simulink model "roll_loop"  (R2019a)
settings: Solver=VariableStepAuto  StartTime=0.0  StopTime=1000  RelTol=1e-3
undefined symbols (not defined in the file): AP, trans_func
settings Model: Creator=nikhil  LastModifiedBy=VTOL_HYD

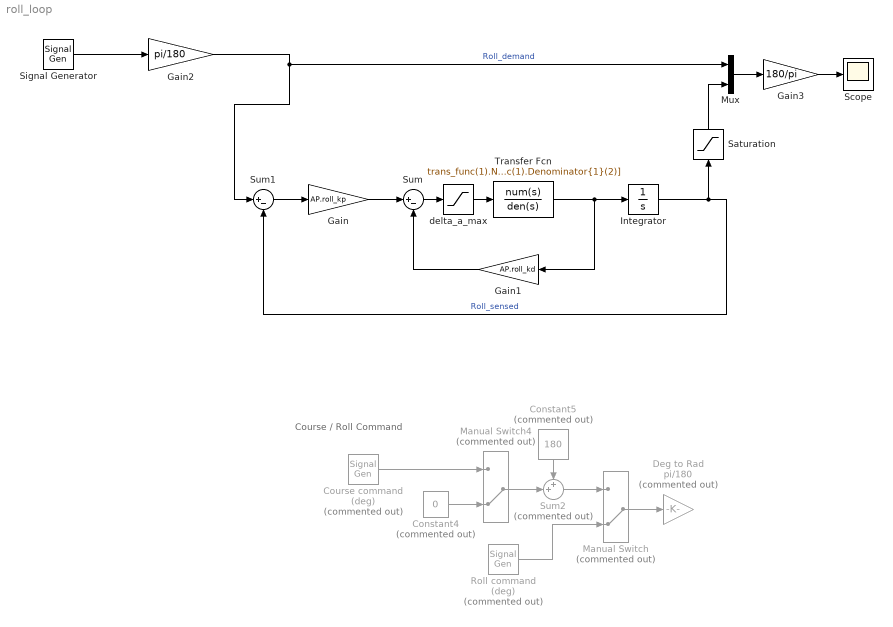
== system roll_loop ==
  note: Course / Roll Command
  Constant4 : Constant  Commented=on  Value=0
  Constant5 : Constant  Commented=on  Value=180
  Course command (deg) : SignalGenerator  Commented=on  WaveForm=square  Amplitude=45  Frequency=.02
  Deg to Rad : Gain  Commented=on  Gain=pi/180
  Gain : Gain  Gain=AP.roll_kp
  Gain1 : Gain  Gain=AP.roll_kd
  Gain2 : Gain  Gain=pi/180
  Gain3 : Gain  Gain=180/pi
  Integrator : Integrator
  Manual Switch : ManualSwitch  Commented=on  CurrentSetting=0
  Manual Switch4 : ManualSwitch  Commented=on  CurrentSetting=0
  Mux : Mux  Inputs=2
  Roll command (deg) : SignalGenerator  Commented=on  Amplitude=180  Frequency=0.1
  Saturation : Saturate  UpperLimit=7  LowerLimit=-7
  Scope : Scope
  Signal Generator : SignalGenerator  Amplitude=45  Frequency=.1  Units=rad/sec
  Sum : Sum  Inputs=|+-
  Sum1 : Sum  Inputs=|+-
  Sum2 : Sum  Commented=on  Inputs=++|
  Transfer Fcn : TransferFcn  Numerator=trans_func(1).Numerator{1}  Denominator=[trans_func(1).Denominator{1}(1), trans_func(1).Denominator{1}(2)]
  delta_a_max : Saturate  UpperLimit=0.785  LowerLimit=-.785
  wires:
  Transfer Fcn/1 -> Gain1/1, Integrator/1
  Integrator/1 -> Sum1/2, Saturation/1  "Roll_sensed"
  Gain1/1 -> Sum/2
  Gain2/1 -> Sum1/1, Mux/1  "Roll_demand"
  Sum1/1 -> Gain/1
  Gain/1 -> Sum/1
  Saturation/1 -> Mux/2
  Signal Generator/1 -> Gain2/1
  Mux/1 -> Gain3/1
  Gain3/1 -> Scope/1
  Sum/1 -> delta_a_max/1
  delta_a_max/1 -> Transfer Fcn/1
  Sum2/1 -> Manual Switch/1
  Constant5/1 -> Sum2/1
  Manual Switch4/1 -> Sum2/2
  Constant4/1 -> Manual Switch4/2
  Roll command (deg)/1 -> Manual Switch/2
  Manual Switch/1 -> Deg to Rad/1
  Course command (deg)/1 -> Manual Switch4/1
